simulink model "BaseModel"  (R2019b)
settings: Solver=VariableStepAuto  StartTime=0.0  StopTime=10  RelTol=1e-3
model workspace (MAT data in the model file):
  K = 184.3
  Ki = 15
  Kp = 5
  g = -9.8
  l = 0.5
  tau = 0.043
settings Model: OrderedModelArguments=off  Creator=gtighe  LastModifiedBy=gtighe

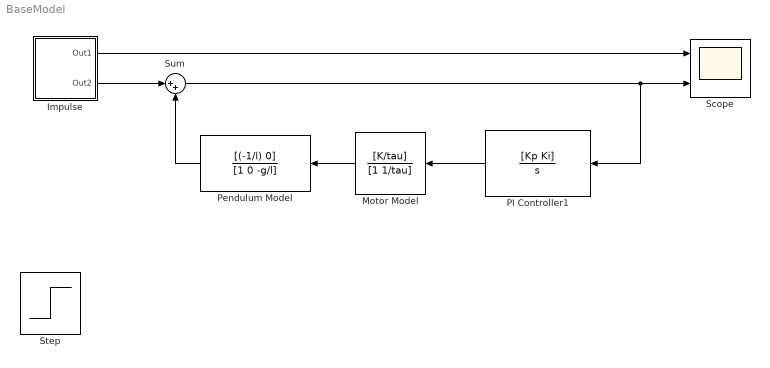
== system BaseModel ==
  Impulse : Subsystem
  Motor Model : TransferFcn  Numerator=[K/tau]  Denominator=[1 1/tau]
  PI Controller1 : TransferFcn  Numerator=[Kp Ki]  Denominator=[1 0]
  Pendulum Model : TransferFcn  Numerator=[(-1/l) 0]  Denominator=[1 0 -g/l]
  Scope : Scope  NumInputPorts=2
  Step : Step  After=200  SampleTime=0
  Sum : Sum  Inputs=|++
  wires:
  Pendulum Model/1 -> Sum/2
  Sum/1 -> Scope/2, PI Controller1/1
  Motor Model/1 -> Pendulum Model/1
  PI Controller1/1 -> Motor Model/1
  Impulse/1(Out1) -> Scope/1
  Impulse/2(Out2) -> Sum/1

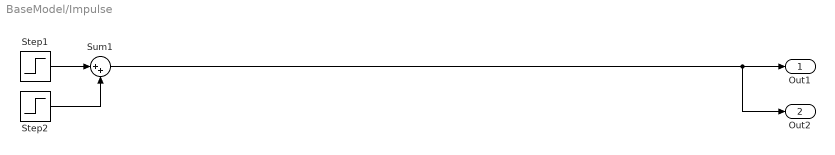
== system BaseModel/Impulse ==
  Step1 : Step  Time=0.25  After=200  SampleTime=0
  Step2 : Step  Time=0.45  After=-200  SampleTime=0
  Sum1 : Sum  Inputs=|++
  Out1 : Outport
  Out2 : Outport  Port=2
  wires:
  Step2/1 -> Sum1/2
  Step1/1 -> Sum1/1
  Sum1/1 -> Out2/1, Out1/1
